simulink model "SRM_2DModel"  (R2025a)
settings: Solver=FixedStepAuto  StartTime=0.0  StopTime=Tsim*4  FixedStep=1e-5  RelTol=1e-3
InitFcn:
  | %thi =12
  | %thf = 56
  | 
  | %Vdc = 96;
values from neighbouring files (symbols this model uses):
  bp_flux_inv = linspace(0, max(flux_matrix(:)), length(u_curr))'    [ParamSweepAndSave.m]    (also in run_simulink_bridge_flux_torq - Copy.m; run_simulink_bridge_flux_torq.m)
  Nc = 10    [ParamSweepAndSave.m]
  Nrpm = 1500    [ParamSweep.m]    (also in ParamSweep1D.m = 2500; ParamSweepAndSave.m)
  table_curr_inv = zeros(length(bp_flux_inv), length(u_pos))    [ParamSweepAndSave.m]    (also in run_simulink_bridge_flux_torq - Copy.m; run_simulink_bridge_flux_torq.m)
  Tsim = pi/4/Nrpm/pi*30    (= 0.005)    [ParamSweep.m]    (also in ParamSweepAndSave.m)
  Vdc = 72    [ParamSweep.m]    (also in ParamSweep1D.m = 96; ParamSweepAndSave.m)
undefined symbols (not defined in the file or in its folder): bp_curr, bp_pos, Ipeak, table_torque
libraries: eeGeneralControl x1, spspowerguiLib x1
settings Model: Creator=PRANJAL  LastModifiedBy=DELL

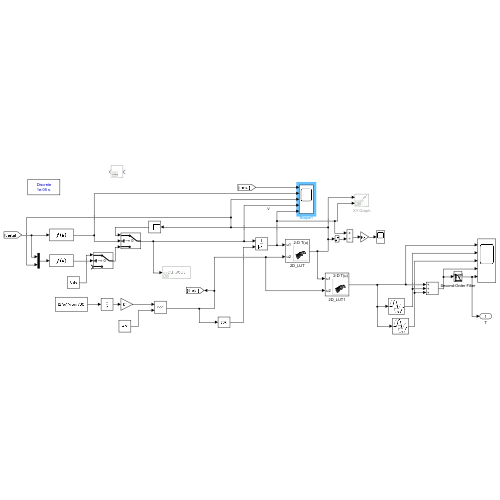
[thumbnail: Simulink's stored preview of the top-level diagram]
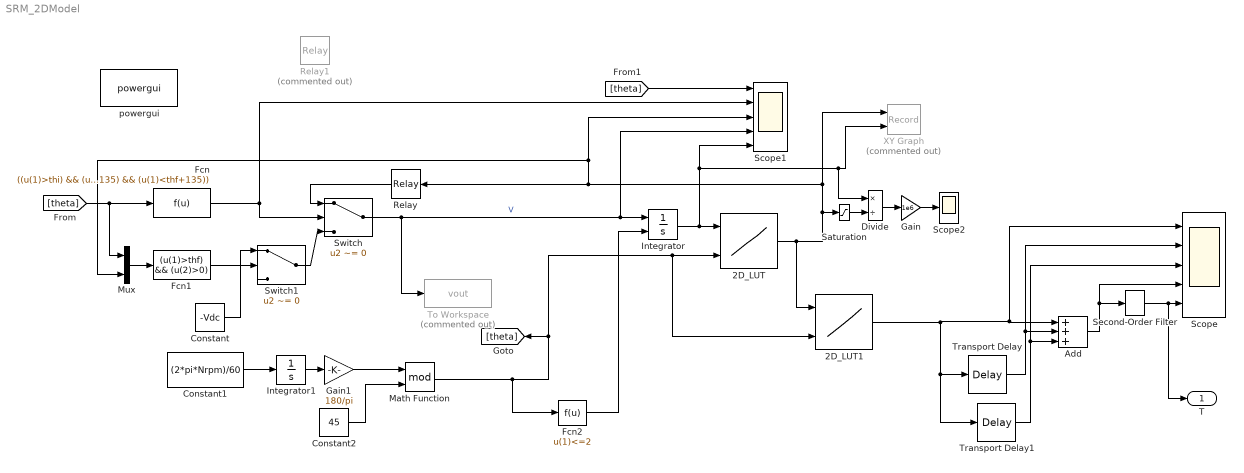
== system SRM_2DModel ==
  2D_LUT : Lookup_n-D  BreakpointsForDimension1=bp_flux_inv*Nc/10  BreakpointsForDimension2=bp_pos-min(bp_pos)  Table=table_curr_inv*10/Nc  InterpMethod=Cubic spline  ExtrapMethod=Cubic spline  InternalRulePriority=Speed  RndMeth=Simplest
      settings: InputPortMap=u0,u1
  2D_LUT1 : Lookup_n-D  BreakpointsForDimension1=bp_curr*10/Nc  BreakpointsForDimension2=bp_pos-min(bp_pos)  Table=table_torque  InterpMethod=Cubic spline  ExtrapMethod=Cubic spline  InternalRulePriority=Speed  RndMeth=Simplest
      settings: InputPortMap=u0,u1
  Add : Sum  Inputs=+++
  Constant : Constant  Value=-Vdc
  Constant1 : Constant  Value=(2*pi*Nrpm)/60
  Constant2 : Constant  Value=45
  Divide : Product  Inputs=*/
  Fcn : Fcn  Expr=((u(1)>thi) && (u(1)<thf)) || ((u(1)>thi+45) && (u(1)<thf+45)) || ((u(1)>thi+90) && (u(1)<thf+90)) || ((u(1)>thi+135) && (u(1)<thf+135))
  Fcn1 : Fcn  Expr=(u(1)>thf) && (u(2)>0)
  Fcn2 : Fcn  Expr=u(1)<=2
  Gain : Gain  Gain=1e6
  Gain1 : Gain  Gain=180/pi
  Integrator : Integrator  ExternalReset=rising
  Integrator1 : Integrator
  Math Function : Math  Operator=mod
  Mux : Mux  Inputs=2
  Relay : Relay  OnSwitchValue=Ipeak*1.05*10/Nc  OffSwitchValue=Ipeak*0.95*10/Nc  OnOutputValue=-Vdc  OffOutputValue=Vdc
  Relay1 : Relay  Commented=on  OnSwitchValue=31*10/Nc  OffSwitchValue=29*10/Nc  OnOutputValue=-Vdc*Nc/10  OffOutputValue=Vdc*Nc/10
  Saturation : Saturate  UpperLimit=1e6  LowerLimit=1
  Scope : Scope  NumInputPorts=5
      settings: ActiveDisplayYMinimum=-102.9035887352433  ActiveDisplayYMaximum=359.2415393407685
  Scope1 : Scope  NumInputPorts=5
      settings: ActiveDisplayYMinimum=-5.6249999999997966  ActiveDisplayYMaximum=50.624999999998181  DataLoggingVariableName=ScopeData3
  Scope2 : Scope
      settings: ActiveDisplayYMinimum=-377.76071773270843  ActiveDisplayYMaximum=199.84645959449085
  Second-Order Filter : eeGeneralControl/Second-Order Filter  FilterType=Low-pass  fn=100  Zeta=0.707  Ts=-1  A0=0  Ph0=0  f0=0  b0=0
      settings: LibrarySourceBlock=ee_sl_lib/General Control/Second-Order Filter
  Switch : Switch  Criteria=u2 ~= 0  Threshold=15  SaturateOnIntegerOverflow=off  InputSameDT=off
  Switch1 : Switch  Criteria=u2 ~= 0  Threshold=15  SaturateOnIntegerOverflow=off  InputSameDT=off
  To Workspace : ToWorkspace  Commented=on  VariableName=vout  SampleTime=-1
  Transport Delay : TransportDelay  DelayTime=Tsim/3  BufferSize=3072
  Transport Delay1 : TransportDelay  DelayTime=2*Tsim/3  BufferSize=3072
  XY Graph : Record  Commented=on  NumPorts=2.0  FileSettingsInternal="{\"entries\":[{\"content\":{\"excelSettings\":{\"content\":{},\"type\":\"Streamout.ExcelSettings\"},\"parquetSettings\":{\"content\":{},\"type\":\"Streamout.ParquetSettings\"}},\"type\":\"Streamout.FileSettingStorage\",\"uuid\":\"\"}],\"packageUris\":[\"http:\\/\\/schema.mathworks.com\\/mf0\\/streamout_blocks\\/R2020a\"],\"version\":\"1.0\"}"  FrameSettings=[0, 0]  Layout=[1 1]  SignalsInternal="{\"entries\":[{\"content\":{},\"type\":\"RecordBlkView.InputSignals\",\"uuid\":\"\"}],\"packageUris\":[\"http:\\/\\/schema.mathworks.com\\/mf0\\/streamout_blocks\\/R2020a\"],\"version\":\"1.0\"}"  VisualizationBindings="{\"xyplotplugin\":{\"info\":[{\"series\":[],\"subplotID\":1}]}}"  CompatibilityTag=XY
  powergui : spspowerguiLib/powergui  Priority=1  SimulationMode=Discrete  SampleTime=10e-6  frequency=60  Iterations=50  frequencyindice=60  Pbase=100e6  ErrMax=1e-4  UnitsV=kV  UnitsW=MW  buscounter=0  FunctionMessages=off  echomessages=off  EnableUseOfTLC=off  CurrentSourceSwitches=off  DisableSnubberDevices=off  DisableRonSwitches=off  DisableVfSwitches=off  DisplayEquations=off  AutomaticDiscreteSolvers=off  SolverType=Tustin/Backward Euler (TBE)  Interpol=off  ExternalGateDelay=off  methode=off  Ts=100  x0status=blocks  SPID=on  SwTol=0  HookPort=off  NonlinearTolerance=1e-4  nMaxIteration=100  ContinueOnMaxIteration=off  RestoreLinks=warning  ResistiveCurrentMeasurement=off  Frange=[0:2:500]  Ylog=off  Xlog=on  ShowGrid=off  save=off  variable=ZData  structure=0  ZoomFFT=off  StartTime=0.0  cycles=1  DisplayStyle=1  fundamental=60  FreqAxis=off  MaxFrequency=1000  frequencyindicesteady=1  RmsSteady=1  display=off
  T : Outport
  wires:
  Add/1 -> Second-Order Filter/1, Scope/4
  Constant1/1 -> Integrator1/1
  Integrator1/1 -> Gain1/1
  Gain1/1 -> Math Function/1
  Constant2/1 -> Math Function/2
  Math Function/1 -> Fcn2/1, [theta], 2D_LUT1/2, 2D_LUT/2
  Transport Delay/1 -> Scope/2, Add/2
  Transport Delay1/1 -> Scope/3, Add/3
  Switch/1 -> Scope1/4, Integrator/1, To Workspace/1  "V"
  Fcn/1 -> Scope1/2, Switch/2
  Relay/1 -> Switch/1
  [theta] -> Mux/1, Fcn/1
  Mux/1 -> Fcn1/1
  Fcn1/1 -> Switch1/2
  Switch1/1 -> Switch/3
  Constant/1 -> Switch1/1
  2D_LUT/1 -> Saturation/1, XY Graph/1, Scope1/3, Mux/2, Relay/1, 2D_LUT1/1
  2D_LUT1/1 -> Add/1, Scope/1, Transport Delay/1, Transport Delay1/1
  [theta] -> Scope1/1
  Second-Order Filter/1 -> T/1, Scope/5
  Fcn2/1 -> Integrator/2
  Integrator/1 -> Scope1/5, Divide/1, XY Graph/2, 2D_LUT/1
  Divide/1 -> Gain/1
  Saturation/1 -> Divide/2
  Gain/1 -> Scope2/1
